simulink model "fsm"  (R2020a)
settings: Solver=VariableStepAuto  StartTime=0.0  StopTime=inf  RelTol=1e-3
settings Model: Creator=Acer  LastModifiedBy=Acer

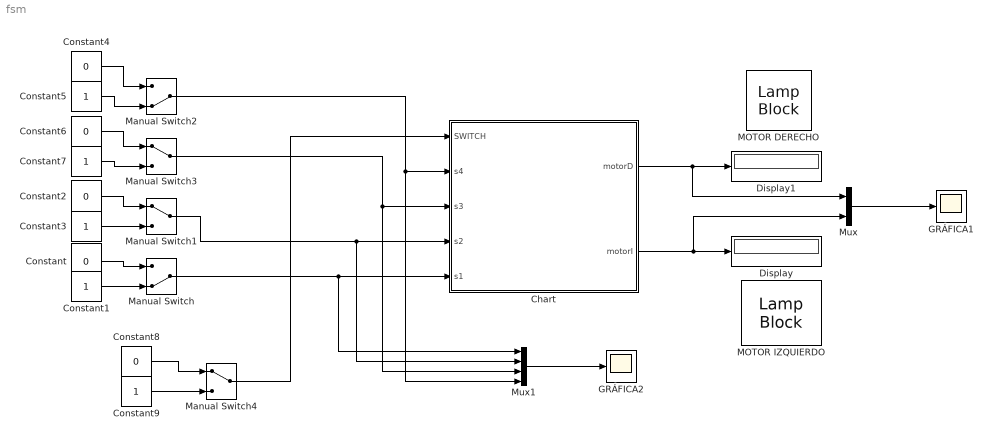
== system fsm ==
  Chart : Stateflow chart  TreatAsAtomicUnit=on
      settings: PortSchema="{\"entries\":[{\"content\":{\"sides\":[{\"content\":{\"connectorIds\":[\"In1\",\"In5\",\"In3\",\"In4\",\"In2\"]},\"type\":\"ConnectorPlacement.EquallySpacedRectSide\",\"uuid\":\"c48cc22e-73b5-437f-8993-9fe880df77c7\"},{\"content\":{\"connectorIds\":[\"Out2\",\"Out1\"],\"side\":\"RIGHT\"},\"type\":\"ConnectorPlacement.EquallySpacedRectSide\",\"uuid\":\"c8cbb8df-0516-4d71-ab05-0b1bf0b46515\"},{\"content\":{\"connectorIds\":[],\"side\":\"TOP\"},\"type\":\"ConnectorPlacement.EquallySpacedRectSide\",\"uuid\":\"fe2c0f7b-0cc0-4864-8066-9d2778e18cac\"}]},\"type\":\"ConnectorPlacement.EquallySpacedConnector\",\"uuid\":\"88afbed0-9649-473f-b301-8b902690c23c\"}],\"packageUris\":[\"http://schema.mathworks.com/mf0/Connector/19700101\"],\"version\":\"1.0\"}"
  Constant{,2,4,6,8} (5 alike) : Constant  Value=0
  Constant{1,3,5,7,9} (5 alike) : Constant
  Display : Display
  Display1 : Display
  GRÁFICA1 : Scope
  GRÁFICA2 : Scope
  MOTOR DERECHO : LampBlock
  MOTOR IZQUIERDO : LampBlock
  Manual Switch : ManualSwitch  CurrentSetting=0
  Manual Switch1 : ManualSwitch
  Manual Switch2 : ManualSwitch  CurrentSetting=0
  Manual Switch3 : ManualSwitch
  Manual Switch4 : ManualSwitch
  Mux : Mux  Inputs=2
  Mux1 : Mux
  wires:
  Constant/1 -> Manual Switch/1
  Constant7/1 -> Manual Switch3/2
  Constant3/1 -> Manual Switch1/2
  Constant6/1 -> Manual Switch3/1
  Constant5/1 -> Manual Switch2/2
  Constant2/1 -> Manual Switch1/1
  Constant1/1 -> Manual Switch/2
  Constant4/1 -> Manual Switch2/1
  Chart/2(motorD) -> Mux/1, Display1/1
  Chart/1(motorI) -> Mux/2, Display/1
  Constant9/1 -> Manual Switch4/2
  Constant8/1 -> Manual Switch4/1
  Manual Switch/1 -> Mux1/1, Chart/2(s1)
  Manual Switch2/1 -> Mux1/4, Chart/5(s4)
  Manual Switch4/1 -> Chart/1(SWITCH)
  Manual Switch1/1 -> Mux1/2, Chart/4(s2)
  Manual Switch3/1 -> Mux1/3, Chart/3(s3)
  Mux/1 -> GRÁFICA1/1
  Mux1/1 -> GRÁFICA2/1

== stateflow chart fsm/Chart ==
  state ON
    state ESTADO_AVANCE
      state ESTADO1AVANCE1
        entry: motorI = 255;
        entry: motorD = 200;
      state ESTADO1AVANCE2
        entry: motorI = 255;
        entry: motorD = 114;
      state ESTADO1AVANCE3
        entry: motorI = 255;
        entry: motorD = 255;
      state ESTADO1AVANCE4
        entry: motorI = 114;
        entry: motorD = 255;
      state ESTADO1AVANCE5
        entry: motorI = 200;
        entry: motorD = 255;
      ESTADO1AVANCE4 -> ESTADO1AVANCE1 [order 4] : [(s1 == 1)&&(s2 == 1)&&(s3 == 0)&&(s4 == 0)]
      ESTADO1AVANCE1 -> ESTADO1AVANCE4 [order 3] : [(s1 == 0)&&(s2 == 1)&&(s3 == 1)&&(s4 == 1)]
      ESTADO1AVANCE2 -> ESTADO1AVANCE5 [order 3] : [(s1 == 0)&&(s2 == 0)&&(s3 == 1)&&(s4 == 1)]
      ESTADO1AVANCE1 -> ESTADO1AVANCE2 [order 1] : [(s1 == 1)&&(s2 == 1)&&(s3 == 1)&&(s4 == 0)]
      ESTADO1AVANCE2 -> ESTADO1AVANCE1 [order 1] : [(s1 == 1)&&(s2 == 1)&&(s3 == 0)&&(s4 == 0)]
      ESTADO1AVANCE5 -> ESTADO1AVANCE2 [order 4] : [(s1 == 1)&&(s2 == 1)&&(s3 == 1)&&(s4 == 0)]
      ESTADO1AVANCE2 -> ESTADO1AVANCE3 [order 2] : [(s1 == 1)&&(s2 == 0)&&(s3 == 0)&&(s4 == 1)]
      ESTADO1AVANCE1 -> ESTADO1AVANCE3 [order 4] : [(s1 == 1)&&(s2 == 0)&&(s3 == 0)&&(s4 == 1)]
      ESTADO1AVANCE3 -> ESTADO1AVANCE2 [order 3] : [(s1 == 1)&&(s2 == 1)&&(s3 == 1)&&(s4 == 0)]
      ESTADO1AVANCE2 -> ESTADO1AVANCE4 [order 4] : [(s1 == 0)&&(s2 == 1)&&(s3 == 1)&&(s4 == 1)]
      ESTADO1AVANCE4 -> ESTADO1AVANCE2 [order 1] : [(s1 == 1)&&(s2 == 1)&&(s3 == 1)&&(s4 == 0)]
      ESTADO1AVANCE1 -> ESTADO1AVANCE5 [order 2] : [(s1 == 0)&&(s2 == 0)&&(s3 == 1)&&(s4 == 1)]
      ESTADO1AVANCE5 -> ESTADO1AVANCE1 [order 1] : [(s1 == 1)&&(s2 == 1)&&(s3 == 0)&&(s4 == 0)]
      ESTADO1AVANCE3 -> ESTADO1AVANCE1 [order 4] : [(s1 == 1)&&(s2 == 1)&&(s3 == 0)&&(s4 == 0)]
      (default) -> ESTADO1AVANCE3
      ESTADO1AVANCE5 -> ESTADO1AVANCE3 [order 2] : [(s1 == 1)&&(s2 == 0)&&(s3 == 0)&&(s4 == 1)]
      ESTADO1AVANCE4 -> ESTADO1AVANCE3 [order 3] : [(s1 == 1)&&(s2 == 0)&&(s3 == 0)&&(s4 == 1)]
      ESTADO1AVANCE3 -> ESTADO1AVANCE5 [order 2] : [(s1 == 0)&&(s2 == 0)&&(s3 == 1)&&(s4 == 1)]
      ESTADO1AVANCE3 -> ESTADO1AVANCE4 [order 1] : [(s1 == 0)&&(s2 == 1)&&(s3 == 1)&&(s4 == 1)]
      ESTADO1AVANCE5 -> ESTADO1AVANCE4 [order 3] : [(s1 == 0)&&(s2 == 1)&&(s3 == 1)&&(s4 == 1)]
      ESTADO1AVANCE4 -> ESTADO1AVANCE5 [order 2] : [(s1 == 0)&&(s2 == 0)&&(s3 == 1)&&(s4 == 1)]
    state ESTADO_RETROCESO
      entry: motorI = 255;
      entry: motorD = 255;
    state ESTADO_GIRO
      state IZQUIERDA
        entry: motorI = 0;
        entry: motorD = 255;
      state DERECHA
        entry: motorI = 255;
        entry: motorD = 0;
      (default) -> IZQUIERDA
      IZQUIERDA -> DERECHA : [(s1 == 1)&&(s2 == 0)&&(s3 == 0)&&(s4 == 0)]
      DERECHA -> IZQUIERDA : [(s1 == 0)&&(s2 == 0)&&(s3 == 0)&&(s4 == 1)]
    state ESTADO_FIN
      entry: motorI = 0;
      entry: motorD = 0;
    ESTADO_AVANCE -> ESTADO_GIRO [order 2] : [((s1 == 0)&&(s2 == 0)&&(s3 == 0)&&(s4 == 1))||((s1 == 1)&&(s2 == 0)&&(s3 == 0)&&(s4 == 0))]
    ESTADO_GIRO -> ESTADO_AVANCE [order 1] : [((s1 == 1)&&(s2 == 0)&&(s3 == 0)&&(s4 == 1))||((s1 == 1)&&(s2 == 1)&&(s3 == 1)&&(s4 == 0))||((s1 == 1)&&(s2 == 1)&&(s3 == 0)&&(s4 == 0))||((s1 == 0)&&(s2 == 0)&&(s3 == 1)&&(s4 == 1))||((s1 == 0)&&(s2 == 1)&&(s3 == 1)&&(s4 == 1))]
    ESTADO_AVANCE -> ESTADO_FIN [order 4] : [(s1 == 0)&&(s2 == 0)&&(s3 == 0)&&(s4 == 0)]
    ESTADO_AVANCE -> ESTADO_RETROCESO [order 3] : [((s1 == 1)&&(s2 == 1)&&(s3 == 1)&&(s4 == 1))]
    ESTADO_RETROCESO -> ESTADO_AVANCE [order 1] : [((s1 == 1)&&(s2 == 0)&&(s3 == 0)&&(s4 == 1))||((s1 == 1)&&(s2 == 1)&&(s3 == 1)&&(s4 == 0))||((s1 == 1)&&(s2 == 1)&&(s3 == 0)&&(s4 == 0))||((s1 == 0)&&(s2 == 0)&&(s3 == 1)&&(s4 == 1))||((s1 == 0)&&(s2 == 1)&&(s3 == 1)&&(s4 == 1))]
    ESTADO_GIRO -> ESTADO_RETROCESO [order 4] : [((s1 == 1)&&(s2 == 1)&&(s3 == 1)&&(s4 == 1))]
    ESTADO_RETROCESO -> ESTADO_GIRO [order 4] : [((s1 == 0)&&(s2 == 0)&&(s3 == 0)&&(s4 == 1))||((s1 == 1)&&(s2 == 0)&&(s3 == 0)&&(s4 == 0))]
    ESTADO_GIRO -> ESTADO_FIN [order 2] : [((s1 == 0)&&(s2 == 0)&&(s3 == 0)&&(s4 == 0))]
    ESTADO_RETROCESO -> ESTADO_FIN [order 2] : [((s1 == 0)&&(s2 == 0)&&(s3 == 0)&&(s4 == 0))]
  state OFF
    entry: s1 == 1;
    entry: s2 == 1;
    entry: s3 == 1;
    entry: s4 == 1;
    entry: motorI == 0;
    entry: motorD == 0;
    exit:
  (default) -> OFF
  OFF -> ESTADO_AVANCE : [SWITCH==1]
  ESTADO_AVANCE -> OFF [order 1] : [SWITCH==0]
  ESTADO_FIN -> OFF : [SWITCH==0]
  ESTADO_RETROCESO -> OFF [order 3] : [SWITCH==0]
  ESTADO_GIRO -> OFF [order 3] : [SWITCH==0]
  data: motorI output; motorD output; SWITCH input; s1 input; s3 input; s2 input; s4 input
